simulink subsystem "LecturaUltrasonidos"  (R2021b)
settings: Solver=VariableStepAuto  StartTime=0.0  StopTime=10.0  RelTol=1e-3
libraries: arduinolib x2
settings Model: Creator=yo  LastModifiedBy=yo

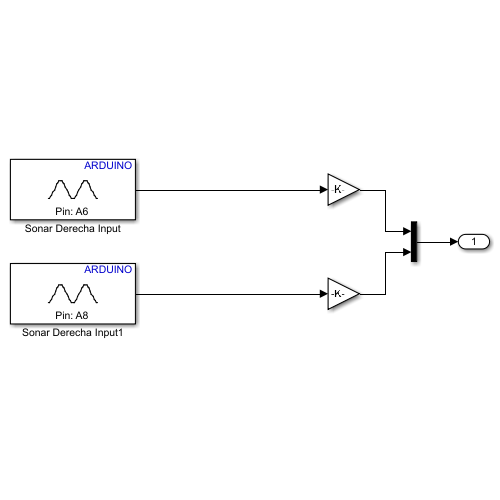
[thumbnail: Simulink's stored preview of the top-level diagram]
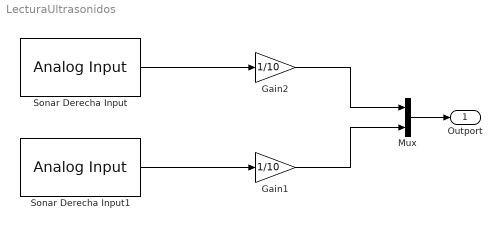
== system LecturaUltrasonidos ==
  Gain1 : Gain  Gain=1/10  OutDataTypeStr=double
  Gain2 : Gain  Gain=1/10  OutDataTypeStr=double
  Mux : Mux  Inputs=2
  Sonar Derecha Input : arduinolib/Analog Input  pinNumber=6  ReadResultsOnly=off  ConversionTriggerSource=Software  ExternalTriggerType=uint32( 0 )  OutputDataType=uint16  EnableConversionCompleteNotify=off  EnableOuputStatus=off  SampleTime=0.01  blockPlatform=arduino
  Sonar Derecha Input1 : arduinolib/Analog Input  pinNumber=7  ReadResultsOnly=off  ConversionTriggerSource=Software  ExternalTriggerType=uint32( 0 )  OutputDataType=uint16  EnableConversionCompleteNotify=off  EnableOuputStatus=off  SampleTime=0.01  blockPlatform=arduino
  Outport : Outport
  wires:
  Gain2/1 -> Mux/1
  Sonar Derecha Input1/1 -> Gain1/1
  Mux/1 -> Outport/1
  Sonar Derecha Input/1 -> Gain2/1
  Gain1/1 -> Mux/2
